simulink model "ldpc"  (R2022b)
settings: Solver=VariableStepAuto  StartTime=0.0  StopTime=10  RelTol=1e-3
model workspace (MAT data in the model file):
  SN = 10
  pcmatrix : object (value not decoded)
libraries: commblkcod2 x2, commdigbbndpm3 x2, commchan3 x1
settings Model: Creator=senol  LastModifiedBy=senol
settings DebuggingCC: ParameterOverflowMsg=none  ParameterUnderflowMsg=error

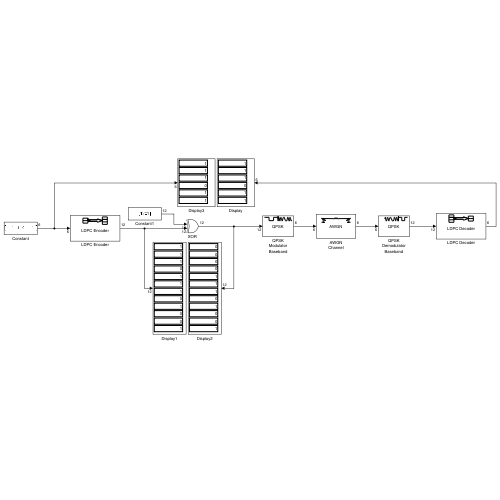
[thumbnail: Simulink's stored preview of the top-level diagram]
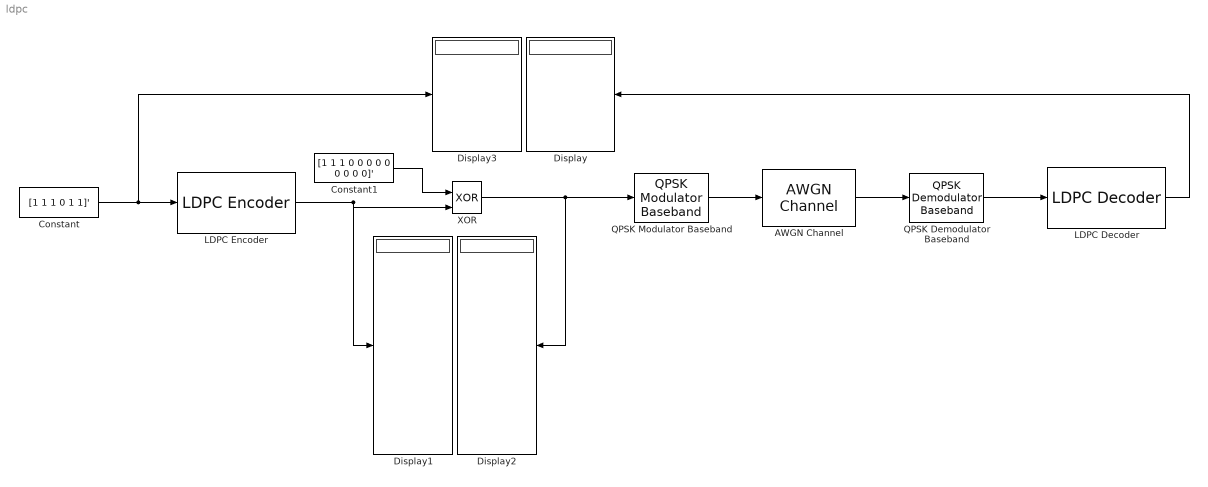
== system ldpc ==
  AWGN Channel : commchan3/AWGN Channel  InputProcessing=Columns as channels (frame based)  seed=67  noiseMode="Signal to noise ratio  (SNR)"  EbNodB=snr  EsNodB=10  SNRdB=SN  bitsPerSym=1  Ps=1  Tsym=1  variance=1
  Constant : Constant  Value=[1 1 1 0 1 1]'  OutDataTypeStr=boolean
  Constant1 : Constant  Value=[1 1 1 0 0 0 0 0 0 0 0 0]'  OutDataTypeStr=boolean
  Display{,1..3} (4 alike) : Display
  LDPC Decoder : commblkcod2/LDPC Decoder  ParityCheckMat=pcmatrix  OutputFmt=Information part  DecisionType=Hard decision  OutputDataType=boolean  NumIter=50  DoParityCheck=off  OutputNumIter=off  OutputFinalChecks=off
  LDPC Encoder : commblkcod2/LDPC Encoder  ParityCheckMat=pcmatrix
  QPSK Demodulator Baseband : commdigbbndpm3/QPSK Demodulator Baseband  OutType=Bit  DecType=Approximate log-likelihood ratio  VarSource=Dialog  Variance=1/10^(SN/10)  Dec=Gray  Ph=pi/4  outDtype1=Inherit via internal rule  outDtype2=Inherit via internal rule  derotateFactorWordLen=16  derotateFactorDataTypeStr=Inherit: Same word length as input  derotateFactorLastDataTypeStr=Inherit: Same word length as input
  QPSK Modulator Baseband : commdigbbndpm3/QPSK Modulator Baseband  InType=Bit  Enc=Gray  Ph=pi/4  outDtype=double  outWordLen=16  outUDDataType=sfix(16)  outFracLenMode=Best precision  outFracLen=15  outDataTypeStr=double  outLastDataTypeStr=double
  XOR : Logic  Operator=XOR  IconShape=distinctive  AllPortsSameDT=off  OutDataTypeStr=boolean
  wires:
  LDPC Encoder/1 -> Display1/1, XOR/2
  Constant/1 -> LDPC Encoder/1, Display3/1
  LDPC Decoder/1 -> Display/1
  Constant1/1 -> XOR/1
  QPSK Demodulator Baseband/1 -> LDPC Decoder/1
  XOR/1 -> QPSK Modulator Baseband/1, Display2/1
  AWGN Channel/1 -> QPSK Demodulator Baseband/1
  QPSK Modulator Baseband/1 -> AWGN Channel/1
